simulink model "Laengsdynamik"  (R2018a)
settings: Solver=FixedStepDiscrete  StartTime=0.0  StopTime=10.0  RelTol=1e-3
values from neighbouring files (symbols this model uses):
  acc_brakes = [ 0 0 0 1 8 8]    [GUI_Fahrdynamik.m]    (also in untitled.m)
  acc_breakpoints = 0:1:5    [GUI_Fahrdynamik.m]    (also in untitled.m)
  Ad = eye(2) + A * dt    [GUI_Fahrdynamik.m]    (also in untitled.m)
  Bd = [dt^2/2;dt]    [GUI_Fahrdynamik.m]    (also in untitled.m)
  C = eye(2)    [GUI_Fahrdynamik.m]    (also in untitled.m)
  chi = h/l    [GUI_Fahrdynamik.m]    (also in untitled.m = 0.178571428571)
  D = [0;0]    [GUI_Fahrdynamik.m]    (also in untitled.m)
  psi = lv/l    [GUI_Fahrdynamik.m]    (also in untitled.m = 0.48)
  x0 = str2double(get(handles.x0, 'String'))    [GUI_Fahrdynamik.m]    (also in untitled.m = [0;30])
  z_bottom = (-((1-psi)/chi))    [GUI_Fahrdynamik.m]    (also in untitled.m = -2.912)
  z_top = (psi/chi)    [GUI_Fahrdynamik.m]    (also in untitled.m = 2.688)
undefined symbols (not defined in the file or in its folder): DiscIntNeverNeededParam
libraries: simulink x1
settings Model: Creator=sebastiankoch  LastModifiedBy=sebastiankoch

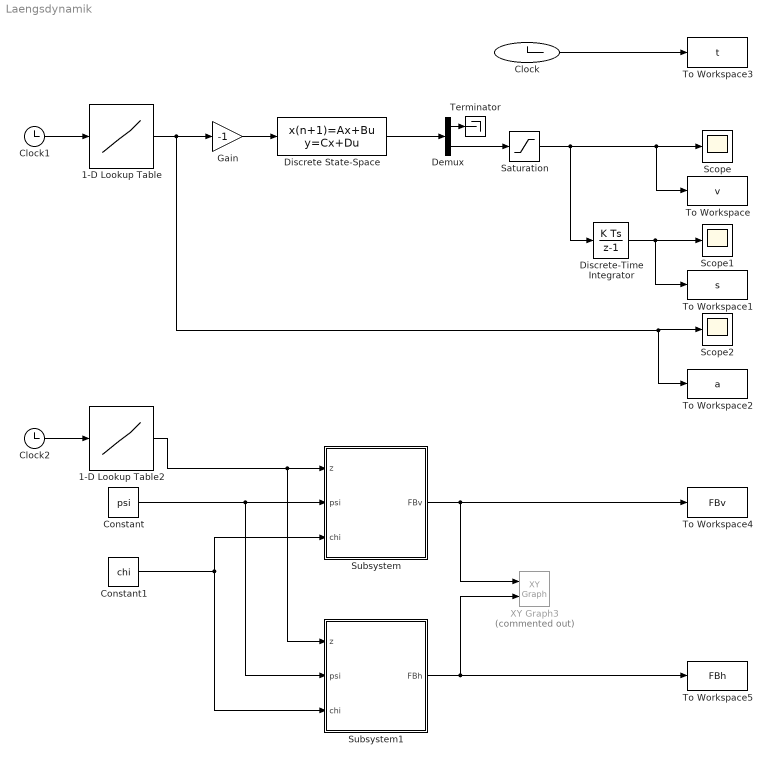
== system Laengsdynamik ==
  1-D Lookup Table : Lookup_n-D  NumberOfTableDimensions=1  BreakpointsForDimension1=acc_breakpoints  Table=acc_brakes  InternalRulePriority=Speed  RndMeth=Simplest  InputSameDT=on
  1-D Lookup Table2 : Lookup_n-D  NumberOfTableDimensions=1  BreakpointsForDimension1=[0 10]  Table=[z_bottom z_top]  InternalRulePriority=Speed  RndMeth=Simplest  InputSameDT=on
  Clock : Clock
  Clock1 : Clock
  Clock2 : Clock
  Constant : Constant  Value=psi
  Constant1 : Constant  Value=chi
  Demux : Demux  Outputs=2
  Discrete State-Space : DiscreteStateSpace  A=Ad  B=Bd  C=C  D=D  InitialCondition=x0  SampleTime=-1
  Discrete-Time Integrator : DiscreteIntegrator  SampleTime=-1  ICPrevOutput=DiscIntNeverNeededParam  ICPrevScaledInput=DiscIntNeverNeededParam
  Gain : Gain  Gain=-1
  Saturation : Saturate  UpperLimit=Inf  LowerLimit=0
  Scope : Scope
  Scope1 : Scope
  Scope2 : Scope
  Subsystem : Subsystem
  Subsystem1 : Subsystem
  Terminator : Terminator
  To Workspace : ToWorkspace  VariableName=v  SampleTime=-1
  To Workspace1 : ToWorkspace  VariableName=s  SampleTime=-1
  To Workspace2 : ToWorkspace  VariableName=a  SampleTime=-1
  To Workspace3 : ToWorkspace  VariableName=t  SampleTime=-1
  To Workspace4 : ToWorkspace  VariableName=FBv  SampleTime=-1
  To Workspace5 : ToWorkspace  VariableName=FBh  SampleTime=-1
  XY Graph3 : simulink/Sinks/XY Graph  Commented=on  xmin=-0.4  xmax=psi/chi  ymin=-((1-psi)/chi)  ymax=psi/chi  st=dt
  wires:
  Gain/1 -> Discrete State-Space/1
  Clock/1 -> To Workspace3/1
  Discrete State-Space/1 -> Demux/1
  Clock1/1 -> 1-D Lookup Table/1
  1-D Lookup Table/1 -> To Workspace2/1, Scope2/1, Gain/1
  Discrete-Time Integrator/1 -> To Workspace1/1, Scope1/1
  Demux/2 -> Saturation/1
  Saturation/1 -> Discrete-Time Integrator/1, Scope/1, To Workspace/1
  Demux/1 -> Terminator/1
  Constant/1 -> Subsystem1/2(psi), Subsystem/2(psi)
  Constant1/1 -> Subsystem/3(chi), Subsystem1/3(chi)
  1-D Lookup Table2/1 -> Subsystem1/1(z), Subsystem/1(z)
  Clock2/1 -> 1-D Lookup Table2/1
  Subsystem1/1(FBh) -> To Workspace5/1, XY Graph3/2
  Subsystem/1(FBv) -> To Workspace4/1, XY Graph3/1

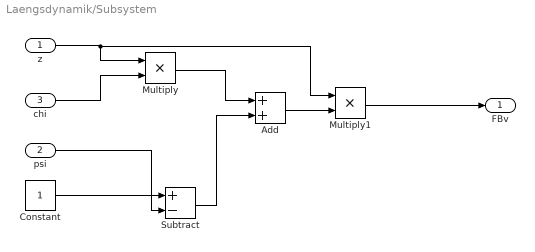
== system Laengsdynamik/Subsystem ==
  z : Inport
  psi : Inport  Port=2
  chi : Inport  Port=3
  Add : Sum
  Constant : Constant
  Multiply : Product
  Multiply1 : Product
  Subtract : Sum  Inputs=+-
  FBv : Outport
  wires:
  Multiply1/1 -> FBv/1
  Constant/1 -> Subtract/1
  psi/1 -> Subtract/2
  chi/1 -> Multiply/2
  z/1 -> Multiply1/1, Multiply/1
  Subtract/1 -> Add/2
  Multiply/1 -> Add/1
  Add/1 -> Multiply1/2

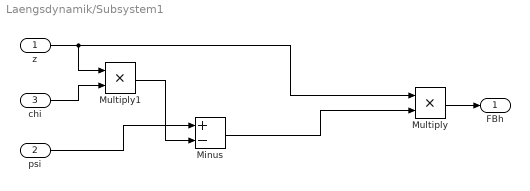
== system Laengsdynamik/Subsystem1 ==
  z : Inport
  psi : Inport  Port=2
  chi : Inport  Port=3
  Minus : Sum  Inputs=+-
  Multiply : Product
  Multiply1 : Product
  FBh : Outport
  wires:
  chi/1 -> Multiply1/2
  z/1 -> Multiply/1, Multiply1/1
  Minus/1 -> Multiply/2
  Multiply/1 -> FBh/1
  psi/1 -> Minus/1
  Multiply1/1 -> Minus/2
